simulink model "motor_tork"  (R2020a)
settings: Solver=VariableStepAuto  StartTime=0.0  StopTime=10.0  RelTol=1e-3
PreLoadFcn:
  | I0 = 2;
InitFcn:
  | init_th1 = 0.0873;
settings Model: Creator=muham  LastModifiedBy=muham
settings SolverCC: AlgebraicLoopSolver=LineSearch

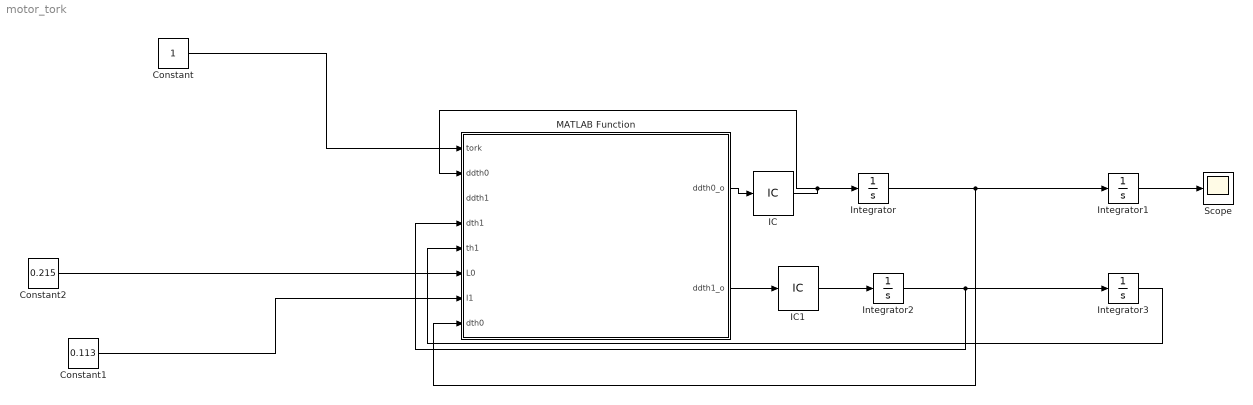
== system motor_tork ==
  Constant : Constant
  Constant1 : Constant  Value=0.113
  Constant2 : Constant  Value=0.215
  IC : InitialCondition  Value=0.00001
  IC1 : InitialCondition  Value=0.00001
  Integrator{,1..3} (4 alike) : Integrator
  MATLAB Function : MATLAB Function  TreatAsAtomicUnit=on
  Scope : Scope
  wires:
  Constant/1 -> MATLAB Function/1(tork)
  Constant1/1 -> MATLAB Function/7(I1)
  Constant2/1 -> MATLAB Function/6(L0)
  MATLAB Function/1(ddth0_o) -> IC/1
  Integrator/1 -> MATLAB Function/8(dth0), Integrator1/1
  Integrator2/1 -> MATLAB Function/4(dth1), Integrator3/1
  MATLAB Function/2(ddth1_o) -> IC1/1
  Integrator3/1 -> MATLAB Function/5(th1)
  IC/1 -> MATLAB Function/2(ddth0), Integrator/1
  Integrator1/1 -> Scope/1
  IC1/1 -> Integrator2/1

== matlab function motor_tork/MATLAB Function ==
  data: tork input; ddth0_o output; ddth0 input; ddth1 input; dth1 input; th1 input; L0 input; I1 input; dth0 input; ddth1_o output
function [ddth0_o, ddth1_o] = motor_src(tork,ddth0, ddth1,dth1,th1,L0,I1,dth0)
m1 = 5.38*10^(-2);
I0 =1.75*10^-2;
J1 = 1.98*10^-4;
g = 9.81;


ddth0_o = (tork-m1*I1*...
    (L0*cos(th1))*ddth1+I1*...
    sin(2*th1)*dth0*dth1-...
    L0*sin(th1)*dth1.^2)/(I0+m1*(L0^2+I1^2*(sin(th1).^2)));
ddth1_o = -( m1*I1*...
    L0*cos(th1)*ddth0-I1*...
     sin(th1)*cos(th1)*dth0.^2-...
    g*sin(th1))/(J1+m1*I1.^2);
end
